simulink subsystem "HEVP1SSC"  (R2022b)
settings: Solver=VariableStepAuto  StartTime=0.0  StopTime=10.0  RelTol=1e-3
undefined symbols (not defined in the file): PlntEM1Inertia, PlntEngInertia
libraries: fl_lib x6, nesl_utility_internal x2
settings Model: Creator=The MathWorks, Inc.  LastModifiedBy=The MathWorks, Inc.

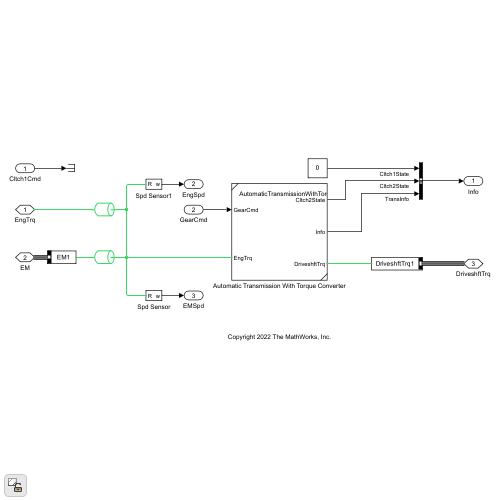
[thumbnail: Simulink's stored preview of the top-level diagram]
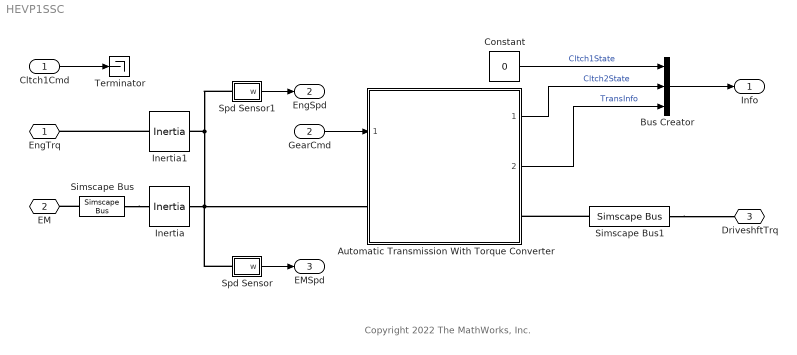
== system HEVP1SSC ==
  note: Copyright 2022 The MathWorks, Inc.
  Cltch1Cmd : Inport
  GearCmd : Inport  Port=2
  Automatic Transmission With Torque Converter : Subsystem  ReferencedSubsystem=AutomaticTransmissionWithTorqueConverterSSC
  Bus Creator : BusCreator  Inputs=3
  Constant : Constant  Value=0  SampleTime=-1
  Inertia : fl_lib/Mechanical/Rotational Elements/Inertia  inertia=PlntEM1Inertia/2 kg*m^2  num_ports=foundation.enum.numPorts2.two  w_specify=off  w_priority=High  w=0 rad/s  w_nominal_specify=off  w_nominal_unit=rad/s  w_nominal_value=1  t_specify=off  t_priority=None  t=0 N*m  t_nominal_specify=off  t_nominal_unit=N*m  t_nominal_value=1
      settings: InternalSimscapePortConfiguration="{\"Bottom\":[],\"Left\":[{\"id\":\"I\",\"label\":\"\",\"type\":\"foundation.mechanical.rotational.rotational\"}],\"Right\":[{\"id\":\"J\",\"label\":\"\",\"type\":\"foundation.mechanical.rotational.rotational\"}],\"Top\":[]}"
  Inertia1 : fl_lib/Mechanical/Rotational Elements/Inertia  inertia=PlntEngInertia/2 kg*m^2  num_ports=foundation.enum.numPorts2.two  w_specify=off  w_priority=High  w=0 rad/s  w_nominal_specify=off  w_nominal_unit=rad/s  w_nominal_value=1  t_specify=off  t_priority=None  t=0 N*m  t_nominal_specify=off  t_nominal_unit=N*m  t_nominal_value=1
      settings: InternalSimscapePortConfiguration="{\"Bottom\":[],\"Left\":[{\"id\":\"I\",\"label\":\"\",\"type\":\"foundation.mechanical.rotational.rotational\"}],\"Right\":[{\"id\":\"J\",\"label\":\"\",\"type\":\"foundation.mechanical.rotational.rotational\"}],\"Top\":[]}"
  Simscape Bus : SimscapeBus  HierarchyStrings=EM1
  Simscape Bus1 : SimscapeBus  HierarchyStrings=DriveshftTrq1
  Spd Sensor : Subsystem
  Spd Sensor1 : Subsystem
  Terminator : Terminator
  EngTrq : PMIOPort  Side=Left
  EM : PMIOPort  Port=2  Side=Left
  DriveshftTrq : PMIOPort  Port=3  Side=Right
  Info : Outport  VectorParamsAs1DForOutWhenUnconnected=off  BusOutputAsStruct=on
  EngSpd : Outport  Port=2  VectorParamsAs1DForOutWhenUnconnected=off  BusOutputAsStruct=on
  EMSpd : Outport  Port=3  VectorParamsAs1DForOutWhenUnconnected=off  BusOutputAsStruct=on
  wires:
  Constant/1 -> Bus Creator/1  "Cltch1State"
  Spd Sensor1/1(w) -> EngSpd/1
  Bus Creator/1 -> Info/1
  Automatic Transmission With Torque Converter/2 -> Bus Creator/3  "TransInfo"
  Automatic Transmission With Torque Converter/1 -> Bus Creator/2  "Cltch2State"
  Cltch1Cmd/1 -> Terminator/1
  Spd Sensor/1(w) -> EMSpd/1
  GearCmd/1 -> Automatic Transmission With Torque Converter/1
  connections:
  Inertia1/RConn1 -- EngTrq/RConn1
  Simscape Bus/RConn1 -- EM/RConn1
  Simscape Bus1/RConn1 -- DriveshftTrq/RConn1
  Simscape Bus1/LConn1 -- Automatic Transmission With Torque Converter/RConn1
  Simscape Bus/LConn1 -- Inertia/RConn1
  Spd Sensor1/LConn1 -- Automatic Transmission With Torque Converter/LConn1 -- Spd Sensor/LConn1 -- Inertia/LConn1 -- Inertia1/LConn1

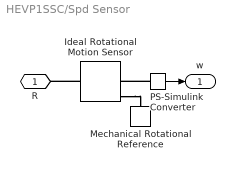
== system HEVP1SSC/Spd Sensor ==
  Ideal Rotational Motion Sensor : fl_lib/Mechanical/Mechanical Sensors/Ideal Rotational Motion Sensor  reference=foundation.enum.MeasurementReference.difference  acceleration_port=false  velocity_port=true  position_port=true  wrap_angle=simscape.enum.onoff.off  offset=0 rad
  Mechanical Rotational Reference : fl_lib/Mechanical/Rotational Elements/Mechanical Rotational Reference
  PS-Simulink Converter : nesl_utility_internal/PS-Simulink Converter  PhysicalDomain=network_engine_domain  SubClassName=ps_output  LeftPortType=input  RightPortType=output  PseudoPeriodic=off  Frequencies=[]  VectorFormat=inherit  Unit=inherit  AffineConversion=off
  R : PMIOPort  Side=Left
  w : Outport
  wires:
  PS-Simulink Converter/1 -> w/1
  connections:
  Ideal Rotational Motion Sensor/RConn1 -- Mechanical Rotational Reference/LConn1
  Ideal Rotational Motion Sensor/LConn1 -- R/RConn1
  PS-Simulink Converter/LConn1 -- Ideal Rotational Motion Sensor/RConn2

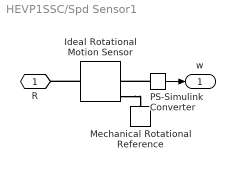
== system HEVP1SSC/Spd Sensor1 ==
  Ideal Rotational Motion Sensor : fl_lib/Mechanical/Mechanical Sensors/Ideal Rotational Motion Sensor  reference=foundation.enum.MeasurementReference.difference  acceleration_port=false  velocity_port=true  position_port=true  wrap_angle=simscape.enum.onoff.off  offset=0 rad
  Mechanical Rotational Reference : fl_lib/Mechanical/Rotational Elements/Mechanical Rotational Reference
  PS-Simulink Converter : nesl_utility_internal/PS-Simulink Converter  PhysicalDomain=network_engine_domain  SubClassName=ps_output  LeftPortType=input  RightPortType=output  PseudoPeriodic=off  Frequencies=[]  VectorFormat=inherit  Unit=inherit  AffineConversion=off
  R : PMIOPort  Side=Left
  w : Outport
  wires:
  PS-Simulink Converter/1 -> w/1
  connections:
  PS-Simulink Converter/LConn1 -- Ideal Rotational Motion Sensor/RConn2
  Ideal Rotational Motion Sensor/LConn1 -- R/RConn1
  Ideal Rotational Motion Sensor/RConn1 -- Mechanical Rotational Reference/LConn1
